simulink model "MVDR_example_hdl_4x4_systolic"  (R2020a)
settings: Solver=FixedStepDiscrete  StartTime=0.0  StopTime=stoptime  RelTol=1e-3
InitFcn:
  | model_init
values from neighbouring files (symbols this model uses):
  BackSubstitutePrototype = fi(0, matrixdivbacksub_dt)    [model_init.m]
  matrixDivDelay = NumberOfCORDICIterations*10 + 86    [model_init.m]
  movavg_bitshift = nextpow2(sqrt(windowSize))    [model_init.m]
  mvdrPipelineDelay = covMatDelay+movAvgDelay+matrixDivDelay+normResponseDelay    [model_init.m]
  numArrayElements = 4    [model_init.m]
  NumberOfCORDICIterations = matrixdivin_dt.WordLength - 1    [model_init.m]
  srcAngles = [20 60]    [model_init.m]
  sv = step(steeringVector,fc,[scanAngle; 0])    [model_init.m]
  Ts = 1/fs    (= 7.8125e-09)    [model_init.m]
  windowSize = 1024    [model_init.m]
libraries: hdlsllib x249, simulink x44, commfilt2 x4, commrfcorlib x3, commsync2 x3, commrflib2 x2, commrandsrc3 x2, phasedtxrxlib x2, commdigbbndcpm2 x1, dspsolvers x1, embreciprocals x1, commdigbbndpm3 x1
(part 6 of 11)

== system MVDR_example_hdl_4x4_systolic/MVDR HDL/Compute Weight Vector/Matrix Left Divide/CORDIC/4x4 Complex CORDIC Matrix Left Divide/Q'B, R 4x4 Complex CORDIC Systolic Array/Leading Complex Row Rotation - 4/Rotate first element to real - 1 ==
  x : Inport
  u : Inport  Port=2
  validIn : Inport  Port=3
  Complex to Real-Imag : ComplexToRealImag
  Complex to Real-Imag1 : ComplexToRealImag
  Delay{4..7,9..10,15} (7 alike) : Delay  DelayLength=1
  Force imaginary part to exactly zero : MATLAB Function  TreatAsAtomicUnit=on
  Inverse CORDIC Gain1 : Subsystem  TreatAsAtomicUnit=on  mask{NumberOfCORDICIterations=NumberOfCORDICIterations}
      mask prompts: NumberOfCORDICIterations "Number of CORDIC Iterations"
      mask Display: disp('1/An')
  Inverse CORDIC Gain2 : Subsystem  TreatAsAtomicUnit=on  mask{NumberOfCORDICIterations=NumberOfCORDICIterations}
      mask prompts: NumberOfCORDICIterations "Number of CORDIC Iterations"
      mask Display: disp('1/An')
  Inverse CORDIC Gain3 : Subsystem  TreatAsAtomicUnit=on  mask{NumberOfCORDICIterations=NumberOfCORDICIterations}
      mask prompts: NumberOfCORDICIterations "Number of CORDIC Iterations"
      mask Display: disp('1/An')
  Inverse CORDIC Gain4 : Subsystem  TreatAsAtomicUnit=on  mask{NumberOfCORDICIterations=NumberOfCORDICIterations}
      mask prompts: NumberOfCORDICIterations "Number of CORDIC Iterations"
      mask Display: disp('1/An')
  "Q'B, R Row Rotations - Real" : Subsystem  TreatAsAtomicUnit=on  mask{NumberOfCORDICIterations=NumberOfCORDICIterations}
      mask prompts: NumberOfCORDICIterations "Number of CORDIC Iterations"
  QR 3rd and 4th Quadrant Compensation : MATLAB Function  TreatAsAtomicUnit=on
  Real-Imag to Complex : RealImagToComplex
  Real-Imag to Complex1 : RealImagToComplex
  State Control : StateControl  StateControl=Synchronous
  Unit Delay Enabled Synchronous{,1..3} (4 alike) : hdlsllib/Discrete/Unit Delay Enabled Synchronous  InitialCondition=0.0  SampleTime=-1
      settings: SourceProductBaseCode=SL
  ValidIn to Ready Logic with Delay : Subsystem
  x' : Outport  VectorParamsAs1DForOutWhenUnconnected=off
  u' : Outport  Port=2  VectorParamsAs1DForOutWhenUnconnected=off
  validOut : Outport  Port=3  VectorParamsAs1DForOutWhenUnconnected=off
  ready : Outport  Port=4  VectorParamsAs1DForOutWhenUnconnected=off
  wires:
  Unit Delay Enabled Synchronous3/1 -> x'/1
  Real-Imag to Complex/1 -> Unit Delay Enabled Synchronous3/1
  Unit Delay Enabled Synchronous2/1 -> u'/1
  Real-Imag to Complex1/1 -> Unit Delay Enabled Synchronous2/1
  Unit Delay Enabled Synchronous1/1 -> Complex to Real-Imag/1
  Unit Delay Enabled Synchronous/1 -> Complex to Real-Imag1/1
  "Q'B, R Row Rotations - Real"/6(ready) -> ValidIn to Ready Logic with Delay/1(readyIn)
  ValidIn to Ready Logic with Delay/1(readyOut) -> ready/1
  Delay15/1 -> validOut/1
  "Q'B, R Row Rotations - Real"/5(validOut) -> Delay15/1, Unit Delay Enabled Synchronous3/2, Unit Delay Enabled Synchronous2/2
  Inverse CORDIC Gain3/1(Out1) -> Real-Imag to Complex1/2
  Inverse CORDIC Gain2/1(Out1) -> Real-Imag to Complex1/1
  Inverse CORDIC Gain1/1(Out1) -> Force imaginary part to exactly zero/1(u)
  Inverse CORDIC Gain4/1(Out1) -> Real-Imag to Complex/1
  Delay10/1 -> "Q'B, R Row Rotations - Real"/5(validIn), ValidIn to Ready Logic with Delay/2(validIn * z^-1)
  validIn/1 -> Delay9/1, Unit Delay Enabled Synchronous1/2, Unit Delay Enabled Synchronous/2
  Delay9/1 -> Delay10/1, ValidIn to Ready Logic with Delay/3(validIn)
  Force imaginary part to exactly zero/1(y) -> Real-Imag to Complex/2
  "Q'B, R Row Rotations - Real"/2(y_out) -> Inverse CORDIC Gain1/1(In1)
  u/1 -> Unit Delay Enabled Synchronous/1
  x/1 -> Unit Delay Enabled Synchronous1/1
  "Q'B, R Row Rotations - Real"/4(v_out) -> Inverse CORDIC Gain3/1(In1)
  "Q'B, R Row Rotations - Real"/3(u_out) -> Inverse CORDIC Gain2/1(In1)
  "Q'B, R Row Rotations - Real"/1(x_out) -> Inverse CORDIC Gain4/1(In1)
  Delay7/1 -> "Q'B, R Row Rotations - Real"/4(v)
  Delay6/1 -> "Q'B, R Row Rotations - Real"/3(u)
  Delay5/1 -> "Q'B, R Row Rotations - Real"/2(y)
  Delay4/1 -> "Q'B, R Row Rotations - Real"/1(x)
  Complex to Real-Imag1/2 -> QR 3rd and 4th Quadrant Compensation/4(v)
  Complex to Real-Imag1/1 -> QR 3rd and 4th Quadrant Compensation/3(u)
  Complex to Real-Imag/2 -> QR 3rd and 4th Quadrant Compensation/2(y)
  Complex to Real-Imag/1 -> QR 3rd and 4th Quadrant Compensation/1(x)
  QR 3rd and 4th Quadrant Compensation/4(v_out) -> Delay7/1
  QR 3rd and 4th Quadrant Compensation/2(y_out) -> Delay5/1
  QR 3rd and 4th Quadrant Compensation/3(u_out) -> Delay6/1
  QR 3rd and 4th Quadrant Compensation/1(x_out) -> Delay4/1

== system MVDR_example_hdl_4x4_systolic/MVDR HDL/Compute Weight Vector/Matrix Left Divide/CORDIC/4x4 Complex CORDIC Matrix Left Divide/Q'B, R 4x4 Complex CORDIC Systolic Array/Leading Complex Row Rotation - 4/ValidIn to Ready Logic ==
  readyIn : Inport
  validIn : Inport  Port=2
  AND : Logic  IconShape=distinctive  AllPortsSameDT=off  OutDataTypeStr=boolean
  NOT : Logic  Operator=NOT  IconShape=distinctive  AllPortsSameDT=off  OutDataTypeStr=boolean
  readyOut : Outport  VectorParamsAs1DForOutWhenUnconnected=off
  wires:
  validIn/1 -> NOT/1
  readyIn/1 -> AND/1
  AND/1 -> readyOut/1
  NOT/1 -> AND/2

== system MVDR_example_hdl_4x4_systolic/MVDR HDL/Compute Weight Vector/Matrix Left Divide/CORDIC/4x4 Complex CORDIC Matrix Left Divide/Q'B, R 4x4 Complex CORDIC Systolic Array/Leading Complex Row Rotation - 4/ValidIn to Ready Logic1 ==
  readyIn : Inport
  validIn : Inport  Port=2
  AND : Logic  IconShape=distinctive  AllPortsSameDT=off  OutDataTypeStr=boolean
  NOT : Logic  Operator=NOT  IconShape=distinctive  AllPortsSameDT=off  OutDataTypeStr=boolean
  readyOut : Outport  VectorParamsAs1DForOutWhenUnconnected=off
  wires:
  validIn/1 -> NOT/1
  readyIn/1 -> AND/1
  AND/1 -> readyOut/1
  NOT/1 -> AND/2

== system MVDR_example_hdl_4x4_systolic/MVDR HDL/Compute Weight Vector/Matrix Left Divide/CORDIC/4x4 Complex CORDIC Matrix Left Divide/Q'B, R 4x4 Complex CORDIC Systolic Array/Rotate first element to real/Inverse CORDIC Gain1 ==
  In1 : Inport
  Inverse CORDIC Gain : Gain  Gain=1/prod(sqrt(1+2.^(-2*(0:double(NumberOfCORDICIterations)-1))))  OutDataTypeStr=Inherit: Same as input
  Out1 : Outport  VectorParamsAs1DForOutWhenUnconnected=off
  wires:
  Inverse CORDIC Gain/1 -> Out1/1
  In1/1 -> Inverse CORDIC Gain/1

== system MVDR_example_hdl_4x4_systolic/MVDR HDL/Compute Weight Vector/Matrix Left Divide/CORDIC/4x4 Complex CORDIC Matrix Left Divide/Q'B, R 4x4 Complex CORDIC Systolic Array/Rotate first element to real/Inverse CORDIC Gain2 ==
  In1 : Inport
  Inverse CORDIC Gain : Gain  Gain=1/prod(sqrt(1+2.^(-2*(0:double(NumberOfCORDICIterations)-1))))  OutDataTypeStr=Inherit: Same as input
  Out1 : Outport  VectorParamsAs1DForOutWhenUnconnected=off
  wires:
  Inverse CORDIC Gain/1 -> Out1/1
  In1/1 -> Inverse CORDIC Gain/1

== system MVDR_example_hdl_4x4_systolic/MVDR HDL/Compute Weight Vector/Matrix Left Divide/CORDIC/4x4 Complex CORDIC Matrix Left Divide/Q'B, R 4x4 Complex CORDIC Systolic Array/Rotate first element to real/Inverse CORDIC Gain3 ==
  In1 : Inport
  Inverse CORDIC Gain : Gain  Gain=1/prod(sqrt(1+2.^(-2*(0:double(NumberOfCORDICIterations)-1))))  OutDataTypeStr=Inherit: Same as input
  Out1 : Outport  VectorParamsAs1DForOutWhenUnconnected=off
  wires:
  Inverse CORDIC Gain/1 -> Out1/1
  In1/1 -> Inverse CORDIC Gain/1

== system MVDR_example_hdl_4x4_systolic/MVDR HDL/Compute Weight Vector/Matrix Left Divide/CORDIC/4x4 Complex CORDIC Matrix Left Divide/Q'B, R 4x4 Complex CORDIC Systolic Array/Rotate first element to real/Inverse CORDIC Gain4 ==
  In1 : Inport
  Inverse CORDIC Gain : Gain  Gain=1/prod(sqrt(1+2.^(-2*(0:double(NumberOfCORDICIterations)-1))))  OutDataTypeStr=Inherit: Same as input
  Out1 : Outport  VectorParamsAs1DForOutWhenUnconnected=off
  wires:
  Inverse CORDIC Gain/1 -> Out1/1
  In1/1 -> Inverse CORDIC Gain/1

== system MVDR_example_hdl_4x4_systolic/MVDR HDL/Compute Weight Vector/Matrix Left Divide/CORDIC/4x4 Complex CORDIC Matrix Left Divide/Q'B, R 4x4 Complex CORDIC Systolic Array/Rotate first element to real/Q'B, R Row Rotations - Real ==
  x : Inport
  y : Inport  Port=2
  u : Inport  Port=3
  v : Inport  Port=4
  validIn : Inport  Port=5
  CORDIC Counter : Subsystem  mask{NumberOfCORDICIterations=NumberOfCORDICIterations}
      mask prompts: NumberOfCORDICIterations "Number of CORDIC Iterations"
  Delay{1..12} (12 alike) : Delay  DelayLength=1
  Delay13 : Delay  DelayLength=1  InitialCondition=true
  MATLAB Function : MATLAB Function  TreatAsAtomicUnit=on
  Same Datatype : Subsystem  TreatAsAtomicUnit=on
  Same Datatype1 : Subsystem  TreatAsAtomicUnit=on
  Same Datatype2 : Subsystem  TreatAsAtomicUnit=on
  Same Datatype3 : Subsystem  TreatAsAtomicUnit=on
  State Control : StateControl  StateControl=Synchronous
  Switch{,1..3} (4 alike) : Switch  Criteria=u2 ~= 0
  x_out : Outport  VectorParamsAs1DForOutWhenUnconnected=off
  y_out : Outport  Port=2  VectorParamsAs1DForOutWhenUnconnected=off
  u_out : Outport  Port=3  VectorParamsAs1DForOutWhenUnconnected=off
  v_out : Outport  Port=4  VectorParamsAs1DForOutWhenUnconnected=off
  validOut : Outport  Port=5  VectorParamsAs1DForOutWhenUnconnected=off
  ready : Outport  Port=6  VectorParamsAs1DForOutWhenUnconnected=off
  wires:
  Delay13/1 -> ready/1
  Delay12/1 -> Delay3/1
  Delay10/1 -> MATLAB Function/5(iteration)
  Delay9/1 -> Switch/2, Switch1/2, Switch2/2, Switch3/2
  Delay8/1 -> Same Datatype2/2(Reference), Switch3/3
  Delay6/1 -> Same Datatype3/2(Reference), Switch2/3
  Delay5/1 -> Same Datatype1/2(Reference), Switch1/3
  Delay4/1 -> Same Datatype/2(Reference), Switch/3
  Delay1/1 -> Same Datatype/1(Data), x_out/1
  Delay2/1 -> Same Datatype1/1(Data), y_out/1
  Delay11/1 -> Same Datatype2/1(Data), v_out/1
  MATLAB Function/1(x_out) -> Delay1/1
  MATLAB Function/2(y_out) -> Delay2/1
  MATLAB Function/3(u_out) -> Delay7/1
  MATLAB Function/4(v_out) -> Delay11/1
  Delay7/1 -> Same Datatype3/1(Data), u_out/1
  Delay3/1 -> validOut/1
  validIn/1 -> CORDIC Counter/1(validIn)
  CORDIC Counter/2(count) -> Delay10/1
  CORDIC Counter/3(last) -> Delay12/1
  CORDIC Counter/4(ready) -> Delay13/1
  Switch/1 -> MATLAB Function/1(x)
  Switch1/1 -> MATLAB Function/2(y)
  Switch2/1 -> MATLAB Function/3(u)
  Switch3/1 -> MATLAB Function/4(v)
  CORDIC Counter/1(count_is_positive) -> Delay9/1
  x/1 -> Delay4/1
  y/1 -> Delay5/1
  u/1 -> Delay6/1
  v/1 -> Delay8/1
  Same Datatype/1(DataOut) -> Switch/1
  Same Datatype1/1(DataOut) -> Switch1/1
  Same Datatype3/1(DataOut) -> Switch2/1
  Same Datatype2/1(DataOut) -> Switch3/1

== system MVDR_example_hdl_4x4_systolic/MVDR HDL/Compute Weight Vector/Matrix Left Divide/CORDIC/4x4 Complex CORDIC Matrix Left Divide/Q'B, R 4x4 Complex CORDIC Systolic Array/Rotate first element to real/ValidIn to Ready Logic with Delay ==
  readyIn : Inport
  validIn * z^-1 : Inport  Port=2
  validIn : Inport  Port=3
  AND : Logic  IconShape=distinctive  AllPortsSameDT=off  OutDataTypeStr=boolean
  AND1 : Logic  IconShape=distinctive  AllPortsSameDT=off  OutDataTypeStr=boolean
  NOT : Logic  Operator=NOT  IconShape=distinctive  AllPortsSameDT=off  OutDataTypeStr=boolean
  NOT1 : Logic  Operator=NOT  IconShape=distinctive  AllPortsSameDT=off  OutDataTypeStr=boolean
  readyOut : Outport  VectorParamsAs1DForOutWhenUnconnected=off
  wires:
  validIn * z^-1/1 -> NOT/1
  validIn/1 -> NOT1/1
  readyIn/1 -> AND/1
  AND1/1 -> readyOut/1
  NOT1/1 -> AND1/2
  NOT/1 -> AND/2
  AND/1 -> AND1/1

== system MVDR_example_hdl_4x4_systolic/MVDR HDL/Compute Weight Vector/Matrix Left Divide/CORDIC/4x4 Complex CORDIC Matrix Left Divide/Back Substitute 4x4 Complex CORDIC/Invert first element - Folded/CORDIC Reciprocal Normalized, Folded/CORDIC Reciprocal Rotations- Folded ==
  x_in : Inport
  validIn : Inport  Port=2
  CORDIC Counter : Subsystem  mask{NumberOfCORDICIterations=NumberOfCORDICIterations}
      mask prompts: NumberOfCORDICIterations "Number of CORDIC Iterations"
  CORDIC Divide Kernel : MATLAB Function  TreatAsAtomicUnit=on
  Delay{1..8} (8 alike) : Delay  DelayLength=1
  Same Datatype1 : Subsystem  TreatAsAtomicUnit=on
  Same Datatype2 : Subsystem  TreatAsAtomicUnit=on
  Same Datatype3 : Subsystem  TreatAsAtomicUnit=on
  z_out : Outport  VectorParamsAs1DForOutWhenUnconnected=off
  validOut : Outport  Port=2  VectorParamsAs1DForOutWhenUnconnected=off
  ready : Outport  Port=3  VectorParamsAs1DForOutWhenUnconnected=off
  wires:
  Delay1/1 -> Same Datatype2/1(Data)
  Delay2/1 -> Same Datatype1/1(Data)
  Delay7/1 -> Same Datatype3/1(Data), z_out/1
  validIn/1 -> CORDIC Counter/1(validIn)
  CORDIC Counter/1(count_is_positive) -> Delay4/1
  CORDIC Counter/2(count) -> Delay5/1
  CORDIC Divide Kernel/1(x_out) -> Delay1/1
  CORDIC Divide Kernel/2(y_out) -> Delay2/1
  CORDIC Divide Kernel/3(z_out) -> Delay7/1
  x_in/1 -> Delay3/1
  Same Datatype1/1(DataOut) -> CORDIC Divide Kernel/2(y_reg)
  Same Datatype3/1(DataOut) -> CORDIC Divide Kernel/3(z_reg)
  CORDIC Counter/3(last) -> Delay6/1
  Same Datatype2/1(DataOut) -> CORDIC Divide Kernel/1(x_reg)
  CORDIC Counter/4(ready) -> Delay8/1
  Delay3/1 -> Same Datatype3/2(Reference), Same Datatype1/2(Reference), Same Datatype2/2(Reference), CORDIC Divide Kernel/4(x_in)
  Delay4/1 -> CORDIC Divide Kernel/5(count_is_positive)
  Delay5/1 -> CORDIC Divide Kernel/6(iteration)
  Delay6/1 -> validOut/1
  Delay8/1 -> ready/1

== system MVDR_example_hdl_4x4_systolic/MVDR HDL/Compute Weight Vector/Matrix Left Divide/CORDIC/4x4 Complex CORDIC Matrix Left Divide/Back Substitute 4x4 Complex CORDIC/Invert first element - Folded/CORDIC Reciprocal Normalized, Folded/Normalizer ==
  u : Inport
  validIn : Inport  Port=2
  Delay{,1..5} (6 alike) : Delay  DelayLength=1
  normalizer_block : MATLAB Function  TreatAsAtomicUnit=on
  u_normalized : Outport  VectorParamsAs1DForOutWhenUnconnected=off
  is_negative : Outport  Port=2  VectorParamsAs1DForOutWhenUnconnected=off
  shift_amount : Outport  Port=3  VectorParamsAs1DForOutWhenUnconnected=off
  validOut : Outport  Port=4  VectorParamsAs1DForOutWhenUnconnected=off
  wires:
  Delay5/1 -> is_negative/1
  normalizer_block/2(is_negative) -> Delay5/1
  Delay4/1 -> validOut/1
  Delay3/1 -> Delay4/1
  validIn/1 -> Delay3/1
  Delay/1 -> normalizer_block/1(u)
  Delay2/1 -> shift_amount/1
  normalizer_block/1(u_normalized) -> Delay1/1
  Delay1/1 -> u_normalized/1
  u/1 -> Delay/1
  normalizer_block/3(shift_amount) -> Delay2/1

== system MVDR_example_hdl_4x4_systolic/MVDR HDL/Compute Weight Vector/Matrix Left Divide/CORDIC/4x4 Complex CORDIC Matrix Left Divide/Back Substitute 4x4 Complex CORDIC/Invert first element - Folded/CORDIC Reciprocal Normalized, Folded/ValidIn to Ready Logic ==
  readyIn : Inport
  validIn : Inport  Port=2
  AND : Logic  IconShape=distinctive  AllPortsSameDT=off  OutDataTypeStr=boolean
  NOT : Logic  Operator=NOT  IconShape=distinctive  AllPortsSameDT=off  OutDataTypeStr=boolean
  readyOut : Outport  VectorParamsAs1DForOutWhenUnconnected=off
  wires:
  validIn/1 -> NOT/1
  readyIn/1 -> AND/1
  AND/1 -> readyOut/1
  NOT/1 -> AND/2

== system MVDR_example_hdl_4x4_systolic/MVDR HDL/Compute Weight Vector/Matrix Left Divide/CORDIC/4x4 Complex CORDIC Matrix Left Divide/Back Substitute 4x4 Complex CORDIC/Invert first element - Folded/CORDIC Reciprocal Normalized, Folded/ValidIn to Ready Logic1 ==
  readyIn : Inport
  validIn : Inport  Port=2
  AND : Logic  IconShape=distinctive  AllPortsSameDT=off  OutDataTypeStr=boolean
  NOT : Logic  Operator=NOT  IconShape=distinctive  AllPortsSameDT=off  OutDataTypeStr=boolean
  readyOut : Outport  VectorParamsAs1DForOutWhenUnconnected=off
  wires:
  validIn/1 -> NOT/1
  readyIn/1 -> AND/1
  AND/1 -> readyOut/1
  NOT/1 -> AND/2

== system MVDR_example_hdl_4x4_systolic/MVDR HDL/Compute Weight Vector/Matrix Left Divide/CORDIC/4x4 Complex CORDIC Matrix Left Divide/Back Substitute 4x4 Complex CORDIC/Invert first element - Folded/CORDIC Reciprocal Normalized, Folded/ValidIn to Ready Logic2 ==
  readyIn : Inport
  validIn : Inport  Port=2
  AND : Logic  IconShape=distinctive  AllPortsSameDT=off  OutDataTypeStr=boolean
  NOT : Logic  Operator=NOT  IconShape=distinctive  AllPortsSameDT=off  OutDataTypeStr=boolean
  readyOut : Outport  VectorParamsAs1DForOutWhenUnconnected=off
  wires:
  validIn/1 -> NOT/1
  readyIn/1 -> AND/1
  AND/1 -> readyOut/1
  NOT/1 -> AND/2

== system MVDR_example_hdl_4x4_systolic/MVDR HDL/Compute Weight Vector/Matrix Left Divide/CORDIC/4x4 Complex CORDIC Matrix Left Divide/Back Substitute 4x4 Complex CORDIC/Invert first element - Folded1/CORDIC Reciprocal Normalized, Folded/CORDIC Reciprocal Rotations- Folded ==
  x_in : Inport
  validIn : Inport  Port=2
  CORDIC Counter : Subsystem  mask{NumberOfCORDICIterations=NumberOfCORDICIterations}
      mask prompts: NumberOfCORDICIterations "Number of CORDIC Iterations"
  CORDIC Divide Kernel : MATLAB Function  TreatAsAtomicUnit=on
  Delay{1..8} (8 alike) : Delay  DelayLength=1
  Same Datatype1 : Subsystem  TreatAsAtomicUnit=on
  Same Datatype2 : Subsystem  TreatAsAtomicUnit=on
  Same Datatype3 : Subsystem  TreatAsAtomicUnit=on
  z_out : Outport  VectorParamsAs1DForOutWhenUnconnected=off
  validOut : Outport  Port=2  VectorParamsAs1DForOutWhenUnconnected=off
  ready : Outport  Port=3  VectorParamsAs1DForOutWhenUnconnected=off
  wires:
  Delay8/1 -> ready/1
  Delay6/1 -> validOut/1
  Delay5/1 -> CORDIC Divide Kernel/6(iteration)
  Delay4/1 -> CORDIC Divide Kernel/5(count_is_positive)
  Delay3/1 -> CORDIC Divide Kernel/4(x_in), Same Datatype2/2(Reference), Same Datatype1/2(Reference), Same Datatype3/2(Reference)
  CORDIC Counter/4(ready) -> Delay8/1
  Same Datatype2/1(DataOut) -> CORDIC Divide Kernel/1(x_reg)
  CORDIC Counter/3(last) -> Delay6/1
  Same Datatype3/1(DataOut) -> CORDIC Divide Kernel/3(z_reg)
  Same Datatype1/1(DataOut) -> CORDIC Divide Kernel/2(y_reg)
  x_in/1 -> Delay3/1
  CORDIC Divide Kernel/3(z_out) -> Delay7/1
  CORDIC Divide Kernel/2(y_out) -> Delay2/1
  CORDIC Divide Kernel/1(x_out) -> Delay1/1
  CORDIC Counter/2(count) -> Delay5/1
  CORDIC Counter/1(count_is_positive) -> Delay4/1
  validIn/1 -> CORDIC Counter/1(validIn)
  Delay7/1 -> z_out/1, Same Datatype3/1(Data)
  Delay2/1 -> Same Datatype1/1(Data)
  Delay1/1 -> Same Datatype2/1(Data)

== system MVDR_example_hdl_4x4_systolic/MVDR HDL/Compute Weight Vector/Matrix Left Divide/CORDIC/4x4 Complex CORDIC Matrix Left Divide/Back Substitute 4x4 Complex CORDIC/Invert first element - Folded1/CORDIC Reciprocal Normalized, Folded/Normalizer ==
  u : Inport
  validIn : Inport  Port=2
  Delay{,1..5} (6 alike) : Delay  DelayLength=1
  normalizer_block : MATLAB Function  TreatAsAtomicUnit=on
  u_normalized : Outport  VectorParamsAs1DForOutWhenUnconnected=off
  is_negative : Outport  Port=2  VectorParamsAs1DForOutWhenUnconnected=off
  shift_amount : Outport  Port=3  VectorParamsAs1DForOutWhenUnconnected=off
  validOut : Outport  Port=4  VectorParamsAs1DForOutWhenUnconnected=off
  wires:
  Delay5/1 -> is_negative/1
  normalizer_block/2(is_negative) -> Delay5/1
  Delay4/1 -> validOut/1
  Delay3/1 -> Delay4/1
  validIn/1 -> Delay3/1
  Delay/1 -> normalizer_block/1(u)
  Delay2/1 -> shift_amount/1
  normalizer_block/1(u_normalized) -> Delay1/1
  Delay1/1 -> u_normalized/1
  u/1 -> Delay/1
  normalizer_block/3(shift_amount) -> Delay2/1

== system MVDR_example_hdl_4x4_systolic/MVDR HDL/Compute Weight Vector/Matrix Left Divide/CORDIC/4x4 Complex CORDIC Matrix Left Divide/Back Substitute 4x4 Complex CORDIC/Invert first element - Folded1/CORDIC Reciprocal Normalized, Folded/ValidIn to Ready Logic ==
  readyIn : Inport
  validIn : Inport  Port=2
  AND : Logic  IconShape=distinctive  AllPortsSameDT=off  OutDataTypeStr=boolean
  NOT : Logic  Operator=NOT  IconShape=distinctive  AllPortsSameDT=off  OutDataTypeStr=boolean
  readyOut : Outport  VectorParamsAs1DForOutWhenUnconnected=off
  wires:
  validIn/1 -> NOT/1
  readyIn/1 -> AND/1
  AND/1 -> readyOut/1
  NOT/1 -> AND/2

== system MVDR_example_hdl_4x4_systolic/MVDR HDL/Compute Weight Vector/Matrix Left Divide/CORDIC/4x4 Complex CORDIC Matrix Left Divide/Back Substitute 4x4 Complex CORDIC/Invert first element - Folded1/CORDIC Reciprocal Normalized, Folded/ValidIn to Ready Logic1 ==
  readyIn : Inport
  validIn : Inport  Port=2
  AND : Logic  IconShape=distinctive  AllPortsSameDT=off  OutDataTypeStr=boolean
  NOT : Logic  Operator=NOT  IconShape=distinctive  AllPortsSameDT=off  OutDataTypeStr=boolean
  readyOut : Outport  VectorParamsAs1DForOutWhenUnconnected=off
  wires:
  validIn/1 -> NOT/1
  readyIn/1 -> AND/1
  AND/1 -> readyOut/1
  NOT/1 -> AND/2

== system MVDR_example_hdl_4x4_systolic/MVDR HDL/Compute Weight Vector/Matrix Left Divide/CORDIC/4x4 Complex CORDIC Matrix Left Divide/Back Substitute 4x4 Complex CORDIC/Invert first element - Folded1/CORDIC Reciprocal Normalized, Folded/ValidIn to Ready Logic2 ==
  readyIn : Inport
  validIn : Inport  Port=2
  AND : Logic  IconShape=distinctive  AllPortsSameDT=off  OutDataTypeStr=boolean
  NOT : Logic  Operator=NOT  IconShape=distinctive  AllPortsSameDT=off  OutDataTypeStr=boolean
  readyOut : Outport  VectorParamsAs1DForOutWhenUnconnected=off
  wires:
  validIn/1 -> NOT/1
  readyIn/1 -> AND/1
  AND/1 -> readyOut/1
  NOT/1 -> AND/2

== system MVDR_example_hdl_4x4_systolic/MVDR HDL/Compute Weight Vector/Matrix Left Divide/CORDIC/4x4 Complex CORDIC Matrix Left Divide/Back Substitute 4x4 Complex CORDIC/Invert first element - Folded2/CORDIC Reciprocal Normalized, Folded/CORDIC Reciprocal Rotations- Folded ==
  x_in : Inport
  validIn : Inport  Port=2
  CORDIC Counter : Subsystem  mask{NumberOfCORDICIterations=NumberOfCORDICIterations}
      mask prompts: NumberOfCORDICIterations "Number of CORDIC Iterations"
  CORDIC Divide Kernel : MATLAB Function  TreatAsAtomicUnit=on
  Delay{1..8} (8 alike) : Delay  DelayLength=1
  Same Datatype1 : Subsystem  TreatAsAtomicUnit=on
  Same Datatype2 : Subsystem  TreatAsAtomicUnit=on
  Same Datatype3 : Subsystem  TreatAsAtomicUnit=on
  z_out : Outport  VectorParamsAs1DForOutWhenUnconnected=off
  validOut : Outport  Port=2  VectorParamsAs1DForOutWhenUnconnected=off
  ready : Outport  Port=3  VectorParamsAs1DForOutWhenUnconnected=off
  wires:
  Delay8/1 -> ready/1
  Delay6/1 -> validOut/1
  Delay5/1 -> CORDIC Divide Kernel/6(iteration)
  Delay4/1 -> CORDIC Divide Kernel/5(count_is_positive)
  Delay3/1 -> CORDIC Divide Kernel/4(x_in), Same Datatype2/2(Reference), Same Datatype1/2(Reference), Same Datatype3/2(Reference)
  CORDIC Counter/4(ready) -> Delay8/1
  Same Datatype2/1(DataOut) -> CORDIC Divide Kernel/1(x_reg)
  CORDIC Counter/3(last) -> Delay6/1
  Same Datatype3/1(DataOut) -> CORDIC Divide Kernel/3(z_reg)
  Same Datatype1/1(DataOut) -> CORDIC Divide Kernel/2(y_reg)
  x_in/1 -> Delay3/1
  CORDIC Divide Kernel/3(z_out) -> Delay7/1
  CORDIC Divide Kernel/2(y_out) -> Delay2/1
  CORDIC Divide Kernel/1(x_out) -> Delay1/1
  CORDIC Counter/2(count) -> Delay5/1
  CORDIC Counter/1(count_is_positive) -> Delay4/1
  validIn/1 -> CORDIC Counter/1(validIn)
  Delay7/1 -> z_out/1, Same Datatype3/1(Data)
  Delay2/1 -> Same Datatype1/1(Data)
  Delay1/1 -> Same Datatype2/1(Data)

== system MVDR_example_hdl_4x4_systolic/MVDR HDL/Compute Weight Vector/Matrix Left Divide/CORDIC/4x4 Complex CORDIC Matrix Left Divide/Back Substitute 4x4 Complex CORDIC/Invert first element - Folded2/CORDIC Reciprocal Normalized, Folded/Normalizer ==
  u : Inport
  validIn : Inport  Port=2
  Delay{,1..5} (6 alike) : Delay  DelayLength=1
  normalizer_block : MATLAB Function  TreatAsAtomicUnit=on
  u_normalized : Outport  VectorParamsAs1DForOutWhenUnconnected=off
  is_negative : Outport  Port=2  VectorParamsAs1DForOutWhenUnconnected=off
  shift_amount : Outport  Port=3  VectorParamsAs1DForOutWhenUnconnected=off
  validOut : Outport  Port=4  VectorParamsAs1DForOutWhenUnconnected=off
  wires:
  Delay5/1 -> is_negative/1
  normalizer_block/2(is_negative) -> Delay5/1
  Delay4/1 -> validOut/1
  Delay3/1 -> Delay4/1
  validIn/1 -> Delay3/1
  Delay/1 -> normalizer_block/1(u)
  Delay2/1 -> shift_amount/1
  normalizer_block/1(u_normalized) -> Delay1/1
  Delay1/1 -> u_normalized/1
  u/1 -> Delay/1
  normalizer_block/3(shift_amount) -> Delay2/1

== system MVDR_example_hdl_4x4_systolic/MVDR HDL/Compute Weight Vector/Matrix Left Divide/CORDIC/4x4 Complex CORDIC Matrix Left Divide/Back Substitute 4x4 Complex CORDIC/Invert first element - Folded2/CORDIC Reciprocal Normalized, Folded/ValidIn to Ready Logic ==
  readyIn : Inport
  validIn : Inport  Port=2
  AND : Logic  IconShape=distinctive  AllPortsSameDT=off  OutDataTypeStr=boolean
  NOT : Logic  Operator=NOT  IconShape=distinctive  AllPortsSameDT=off  OutDataTypeStr=boolean
  readyOut : Outport  VectorParamsAs1DForOutWhenUnconnected=off
  wires:
  validIn/1 -> NOT/1
  readyIn/1 -> AND/1
  AND/1 -> readyOut/1
  NOT/1 -> AND/2

== system MVDR_example_hdl_4x4_systolic/MVDR HDL/Compute Weight Vector/Matrix Left Divide/CORDIC/4x4 Complex CORDIC Matrix Left Divide/Back Substitute 4x4 Complex CORDIC/Invert first element - Folded2/CORDIC Reciprocal Normalized, Folded/ValidIn to Ready Logic1 ==
  readyIn : Inport
  validIn : Inport  Port=2
  AND : Logic  IconShape=distinctive  AllPortsSameDT=off  OutDataTypeStr=boolean
  NOT : Logic  Operator=NOT  IconShape=distinctive  AllPortsSameDT=off  OutDataTypeStr=boolean
  readyOut : Outport  VectorParamsAs1DForOutWhenUnconnected=off
  wires:
  validIn/1 -> NOT/1
  readyIn/1 -> AND/1
  AND/1 -> readyOut/1
  NOT/1 -> AND/2

== system MVDR_example_hdl_4x4_systolic/MVDR HDL/Compute Weight Vector/Matrix Left Divide/CORDIC/4x4 Complex CORDIC Matrix Left Divide/Back Substitute 4x4 Complex CORDIC/Invert first element - Folded2/CORDIC Reciprocal Normalized, Folded/ValidIn to Ready Logic2 ==
  readyIn : Inport
  validIn : Inport  Port=2
  AND : Logic  IconShape=distinctive  AllPortsSameDT=off  OutDataTypeStr=boolean
  NOT : Logic  Operator=NOT  IconShape=distinctive  AllPortsSameDT=off  OutDataTypeStr=boolean
  readyOut : Outport  VectorParamsAs1DForOutWhenUnconnected=off
  wires:
  validIn/1 -> NOT/1
  readyIn/1 -> AND/1
  AND/1 -> readyOut/1
  NOT/1 -> AND/2

== system MVDR_example_hdl_4x4_systolic/MVDR HDL/Compute Weight Vector/Matrix Left Divide/CORDIC/4x4 Complex CORDIC Matrix Left Divide/Back Substitute 4x4 Complex CORDIC/Invert first element - Folded3/CORDIC Reciprocal Normalized, Folded/CORDIC Reciprocal Rotations- Folded ==
  x_in : Inport
  validIn : Inport  Port=2
  CORDIC Counter : Subsystem  mask{NumberOfCORDICIterations=NumberOfCORDICIterations}
      mask prompts: NumberOfCORDICIterations "Number of CORDIC Iterations"
  CORDIC Divide Kernel : MATLAB Function  TreatAsAtomicUnit=on
  Delay{1..8} (8 alike) : Delay  DelayLength=1
  Same Datatype1 : Subsystem  TreatAsAtomicUnit=on
  Same Datatype2 : Subsystem  TreatAsAtomicUnit=on
  Same Datatype3 : Subsystem  TreatAsAtomicUnit=on
  z_out : Outport  VectorParamsAs1DForOutWhenUnconnected=off
  validOut : Outport  Port=2  VectorParamsAs1DForOutWhenUnconnected=off
  ready : Outport  Port=3  VectorParamsAs1DForOutWhenUnconnected=off
  wires:
  Delay8/1 -> ready/1
  Delay6/1 -> validOut/1
  Delay5/1 -> CORDIC Divide Kernel/6(iteration)
  Delay4/1 -> CORDIC Divide Kernel/5(count_is_positive)
  Delay3/1 -> CORDIC Divide Kernel/4(x_in), Same Datatype2/2(Reference), Same Datatype1/2(Reference), Same Datatype3/2(Reference)
  CORDIC Counter/4(ready) -> Delay8/1
  Same Datatype2/1(DataOut) -> CORDIC Divide Kernel/1(x_reg)
  CORDIC Counter/3(last) -> Delay6/1
  Same Datatype3/1(DataOut) -> CORDIC Divide Kernel/3(z_reg)
  Same Datatype1/1(DataOut) -> CORDIC Divide Kernel/2(y_reg)
  x_in/1 -> Delay3/1
  CORDIC Divide Kernel/3(z_out) -> Delay7/1
  CORDIC Divide Kernel/2(y_out) -> Delay2/1
  CORDIC Divide Kernel/1(x_out) -> Delay1/1
  CORDIC Counter/2(count) -> Delay5/1
  CORDIC Counter/1(count_is_positive) -> Delay4/1
  validIn/1 -> CORDIC Counter/1(validIn)
  Delay7/1 -> z_out/1, Same Datatype3/1(Data)
  Delay2/1 -> Same Datatype1/1(Data)
  Delay1/1 -> Same Datatype2/1(Data)

== system MVDR_example_hdl_4x4_systolic/MVDR HDL/Compute Weight Vector/Matrix Left Divide/CORDIC/4x4 Complex CORDIC Matrix Left Divide/Back Substitute 4x4 Complex CORDIC/Invert first element - Folded3/CORDIC Reciprocal Normalized, Folded/Normalizer ==
  u : Inport
  validIn : Inport  Port=2
  Delay{,1..5} (6 alike) : Delay  DelayLength=1
  normalizer_block : MATLAB Function  TreatAsAtomicUnit=on
  u_normalized : Outport  VectorParamsAs1DForOutWhenUnconnected=off
  is_negative : Outport  Port=2  VectorParamsAs1DForOutWhenUnconnected=off
  shift_amount : Outport  Port=3  VectorParamsAs1DForOutWhenUnconnected=off
  validOut : Outport  Port=4  VectorParamsAs1DForOutWhenUnconnected=off
  wires:
  Delay5/1 -> is_negative/1
  normalizer_block/2(is_negative) -> Delay5/1
  Delay4/1 -> validOut/1
  Delay3/1 -> Delay4/1
  validIn/1 -> Delay3/1
  Delay/1 -> normalizer_block/1(u)
  Delay2/1 -> shift_amount/1
  normalizer_block/1(u_normalized) -> Delay1/1
  Delay1/1 -> u_normalized/1
  u/1 -> Delay/1
  normalizer_block/3(shift_amount) -> Delay2/1

== system MVDR_example_hdl_4x4_systolic/MVDR HDL/Compute Weight Vector/Matrix Left Divide/CORDIC/4x4 Complex CORDIC Matrix Left Divide/Back Substitute 4x4 Complex CORDIC/Invert first element - Folded3/CORDIC Reciprocal Normalized, Folded/ValidIn to Ready Logic ==
  readyIn : Inport
  validIn : Inport  Port=2
  AND : Logic  IconShape=distinctive  AllPortsSameDT=off  OutDataTypeStr=boolean
  NOT : Logic  Operator=NOT  IconShape=distinctive  AllPortsSameDT=off  OutDataTypeStr=boolean
  readyOut : Outport  VectorParamsAs1DForOutWhenUnconnected=off
  wires:
  validIn/1 -> NOT/1
  readyIn/1 -> AND/1
  AND/1 -> readyOut/1
  NOT/1 -> AND/2

== system MVDR_example_hdl_4x4_systolic/MVDR HDL/Compute Weight Vector/Matrix Left Divide/CORDIC/4x4 Complex CORDIC Matrix Left Divide/Back Substitute 4x4 Complex CORDIC/Invert first element - Folded3/CORDIC Reciprocal Normalized, Folded/ValidIn to Ready Logic1 ==
  readyIn : Inport
  validIn : Inport  Port=2
  AND : Logic  IconShape=distinctive  AllPortsSameDT=off  OutDataTypeStr=boolean
  NOT : Logic  Operator=NOT  IconShape=distinctive  AllPortsSameDT=off  OutDataTypeStr=boolean
  readyOut : Outport  VectorParamsAs1DForOutWhenUnconnected=off
  wires:
  validIn/1 -> NOT/1
  readyIn/1 -> AND/1
  AND/1 -> readyOut/1
  NOT/1 -> AND/2

== system MVDR_example_hdl_4x4_systolic/MVDR HDL/Compute Weight Vector/Matrix Left Divide/CORDIC/4x4 Complex CORDIC Matrix Left Divide/Back Substitute 4x4 Complex CORDIC/Invert first element - Folded3/CORDIC Reciprocal Normalized, Folded/ValidIn to Ready Logic2 ==
  readyIn : Inport
  validIn : Inport  Port=2
  AND : Logic  IconShape=distinctive  AllPortsSameDT=off  OutDataTypeStr=boolean
  NOT : Logic  Operator=NOT  IconShape=distinctive  AllPortsSameDT=off  OutDataTypeStr=boolean
  readyOut : Outport  VectorParamsAs1DForOutWhenUnconnected=off
  wires:
  validIn/1 -> NOT/1
  readyIn/1 -> AND/1
  AND/1 -> readyOut/1
  NOT/1 -> AND/2

== system MVDR_example_hdl_4x4_systolic/MVDR HDL/Compute Weight Vector/Matrix Left Divide/CORDIC/4x4 Complex CORDIC Matrix Left Divide/Q'B, R 4x4 Complex CORDIC Systolic Array/Complex Row Rotation with real pivots/Q'B, R Row Rotations - Complex/CORDIC Counter ==
  validIn : Inport
  Compare To Constant : simulink/Logic and Bit Operations/Compare To Constant  relop===  const=NumberOfCORDICIterations-1  OutDataTypeStr=boolean
  Compare To Zero : simulink/Logic and Bit Operations/Compare To Zero  relop=>  OutDataTypeStr=boolean
  HDL Counter1 : hdlsllib/Sources/HDL Counter  CountType=Count limited  CountInit=0  CountStep=1  CountMax=NumberOfCORDICIterations-1  CountFromType=Initial value  CountFrom=0  CountResetPort=off  CountLoadPort=off  CountEnbPort=on  CountDirPort=off  CountDataType=Unsigned  CountWordLen=nextpow2(NumberOfCORDICIterations)  CountFracLen=0  CountSampTime=1
  OR : Logic  Operator=OR  IconShape=distinctive  AllPortsSameDT=off  OutDataTypeStr=boolean
  SR_latch : Subsystem
  State Control : StateControl  StateControl=Synchronous
  ValidIn to Ready Logic : Subsystem
  count_is_positive : Outport  VectorParamsAs1DForOutWhenUnconnected=off
  count : Outport  Port=2  VectorParamsAs1DForOutWhenUnconnected=off
  last : Outport  Port=3  VectorParamsAs1DForOutWhenUnconnected=off
  ready : Outport  Port=4  VectorParamsAs1DForOutWhenUnconnected=off
  wires:
  ValidIn to Ready Logic/1(readyOut) -> ready/1
  SR_latch/1(Q) -> ValidIn to Ready Logic/1(readyIn)  "ready"
  validIn/1 -> OR/2, SR_latch/2(R), ValidIn to Ready Logic/2(validIn)
  Compare To Constant/1 -> last/1, SR_latch/1(S)
  Compare To Zero/1 -> OR/1, count_is_positive/1
  OR/1 -> HDL Counter1/1
  HDL Counter1/1 -> Compare To Constant/1, count/1, Compare To Zero/1  "count"

== system MVDR_example_hdl_4x4_systolic/MVDR HDL/Compute Weight Vector/Matrix Left Divide/CORDIC/4x4 Complex CORDIC Matrix Left Divide/Q'B, R 4x4 Complex CORDIC Systolic Array/Complex Row Rotation with real pivots/Q'B, R Row Rotations - Complex/Same Datatype ==
  Data : Inport
  Reference : Inport  Port=2
  Data Type Duplicate : DataTypeDuplicate
  DataOut : Outport  VectorParamsAs1DForOutWhenUnconnected=off
  wires:
  Data/1 -> Data Type Duplicate/1, DataOut/1
  Reference/1 -> Data Type Duplicate/2

== system MVDR_example_hdl_4x4_systolic/MVDR HDL/Compute Weight Vector/Matrix Left Divide/CORDIC/4x4 Complex CORDIC Matrix Left Divide/Q'B, R 4x4 Complex CORDIC Systolic Array/Complex Row Rotation with real pivots/Q'B, R Row Rotations - Complex/Same Datatype1 ==
  Data : Inport
  Reference : Inport  Port=2
  Data Type Duplicate : DataTypeDuplicate
  DataOut : Outport  VectorParamsAs1DForOutWhenUnconnected=off
  wires:
  Data/1 -> Data Type Duplicate/1, DataOut/1
  Reference/1 -> Data Type Duplicate/2

== system MVDR_example_hdl_4x4_systolic/MVDR HDL/Compute Weight Vector/Matrix Left Divide/CORDIC/4x4 Complex CORDIC Matrix Left Divide/Q'B, R 4x4 Complex CORDIC Systolic Array/Complex Row Rotation with real pivots/Q'B, R Row Rotations - Complex/Same Datatype2 ==
  Data : Inport
  Reference : Inport  Port=2
  Data Type Duplicate : DataTypeDuplicate
  DataOut : Outport  VectorParamsAs1DForOutWhenUnconnected=off
  wires:
  Data/1 -> Data Type Duplicate/1, DataOut/1
  Reference/1 -> Data Type Duplicate/2

== system MVDR_example_hdl_4x4_systolic/MVDR HDL/Compute Weight Vector/Matrix Left Divide/CORDIC/4x4 Complex CORDIC Matrix Left Divide/Q'B, R 4x4 Complex CORDIC Systolic Array/Complex Row Rotation with real pivots/Q'B, R Row Rotations - Complex/Same Datatype3 ==
  Data : Inport
  Reference : Inport  Port=2
  Data Type Duplicate : DataTypeDuplicate
  DataOut : Outport  VectorParamsAs1DForOutWhenUnconnected=off
  wires:
  Data/1 -> Data Type Duplicate/1, DataOut/1
  Reference/1 -> Data Type Duplicate/2

== system MVDR_example_hdl_4x4_systolic/MVDR HDL/Compute Weight Vector/Matrix Left Divide/CORDIC/4x4 Complex CORDIC Matrix Left Divide/Q'B, R 4x4 Complex CORDIC Systolic Array/Complex Row Rotation 1/Q'B, R Row Rotations - Complex - Folded/CORDIC Counter ==
  validIn : Inport
  Compare To Constant : simulink/Logic and Bit Operations/Compare To Constant  relop===  const=NumberOfCORDICIterations-1  OutDataTypeStr=boolean
  Compare To Zero : simulink/Logic and Bit Operations/Compare To Zero  relop=>  OutDataTypeStr=boolean
  HDL Counter1 : hdlsllib/Sources/HDL Counter  CountType=Count limited  CountInit=0  CountStep=1  CountMax=NumberOfCORDICIterations-1  CountFromType=Initial value  CountFrom=0  CountResetPort=off  CountLoadPort=off  CountEnbPort=on  CountDirPort=off  CountDataType=Unsigned  CountWordLen=nextpow2(NumberOfCORDICIterations)  CountFracLen=0  CountSampTime=1
  OR : Logic  Operator=OR  IconShape=distinctive  AllPortsSameDT=off  OutDataTypeStr=boolean
  SR_latch : Subsystem
  State Control : StateControl  StateControl=Synchronous
  ValidIn to Ready Logic : Subsystem
  count_is_positive : Outport  VectorParamsAs1DForOutWhenUnconnected=off
  count : Outport  Port=2  VectorParamsAs1DForOutWhenUnconnected=off
  last : Outport  Port=3  VectorParamsAs1DForOutWhenUnconnected=off
  ready : Outport  Port=4  VectorParamsAs1DForOutWhenUnconnected=off
  wires:
  ValidIn to Ready Logic/1(readyOut) -> ready/1
  SR_latch/1(Q) -> ValidIn to Ready Logic/1(readyIn)  "ready"
  validIn/1 -> OR/2, SR_latch/2(R), ValidIn to Ready Logic/2(validIn)
  Compare To Constant/1 -> last/1, SR_latch/1(S)
  Compare To Zero/1 -> OR/1, count_is_positive/1
  OR/1 -> HDL Counter1/1
  HDL Counter1/1 -> Compare To Constant/1, count/1, Compare To Zero/1  "count"

== system MVDR_example_hdl_4x4_systolic/MVDR HDL/Compute Weight Vector/Matrix Left Divide/CORDIC/4x4 Complex CORDIC Matrix Left Divide/Q'B, R 4x4 Complex CORDIC Systolic Array/Complex Row Rotation 1/Q'B, R Row Rotations - Complex - Folded/Same Datatype ==
  Data : Inport
  Reference : Inport  Port=2
  Data Type Duplicate : DataTypeDuplicate
  DataOut : Outport  VectorParamsAs1DForOutWhenUnconnected=off
  wires:
  Data/1 -> Data Type Duplicate/1, DataOut/1
  Reference/1 -> Data Type Duplicate/2

== system MVDR_example_hdl_4x4_systolic/MVDR HDL/Compute Weight Vector/Matrix Left Divide/CORDIC/4x4 Complex CORDIC Matrix Left Divide/Q'B, R 4x4 Complex CORDIC Systolic Array/Complex Row Rotation 1/Q'B, R Row Rotations - Complex - Folded/Same Datatype1 ==
  Data : Inport
  Reference : Inport  Port=2
  Data Type Duplicate : DataTypeDuplicate
  DataOut : Outport  VectorParamsAs1DForOutWhenUnconnected=off
  wires:
  Data/1 -> Data Type Duplicate/1, DataOut/1
  Reference/1 -> Data Type Duplicate/2

== system MVDR_example_hdl_4x4_systolic/MVDR HDL/Compute Weight Vector/Matrix Left Divide/CORDIC/4x4 Complex CORDIC Matrix Left Divide/Q'B, R 4x4 Complex CORDIC Systolic Array/Complex Row Rotation 1/Q'B, R Row Rotations - Complex - Folded/Same Datatype2 ==
  Data : Inport
  Reference : Inport  Port=2
  Data Type Duplicate : DataTypeDuplicate
  DataOut : Outport  VectorParamsAs1DForOutWhenUnconnected=off
  wires:
  Data/1 -> Data Type Duplicate/1, DataOut/1
  Reference/1 -> Data Type Duplicate/2

== system MVDR_example_hdl_4x4_systolic/MVDR HDL/Compute Weight Vector/Matrix Left Divide/CORDIC/4x4 Complex CORDIC Matrix Left Divide/Q'B, R 4x4 Complex CORDIC Systolic Array/Complex Row Rotation 1/Q'B, R Row Rotations - Complex - Folded/Same Datatype3 ==
  Data : Inport
  Reference : Inport  Port=2
  Data Type Duplicate : DataTypeDuplicate
  DataOut : Outport  VectorParamsAs1DForOutWhenUnconnected=off
  wires:
  Data/1 -> Data Type Duplicate/1, DataOut/1
  Reference/1 -> Data Type Duplicate/2

== system MVDR_example_hdl_4x4_systolic/MVDR HDL/Compute Weight Vector/Matrix Left Divide/CORDIC/4x4 Complex CORDIC Matrix Left Divide/Q'B, R 4x4 Complex CORDIC Systolic Array/Complex Row Rotation 1/Rotate first element to real - Folded/Inverse CORDIC Gain1 ==
  In1 : Inport
  Inverse CORDIC Gain : Gain  Gain=1/prod(sqrt(1+2.^(-2*(0:double(NumberOfCORDICIterations)-1))))  OutDataTypeStr=Inherit: Same as input
  Out1 : Outport  VectorParamsAs1DForOutWhenUnconnected=off
  wires:
  Inverse CORDIC Gain/1 -> Out1/1
  In1/1 -> Inverse CORDIC Gain/1

== system MVDR_example_hdl_4x4_systolic/MVDR HDL/Compute Weight Vector/Matrix Left Divide/CORDIC/4x4 Complex CORDIC Matrix Left Divide/Q'B, R 4x4 Complex CORDIC Systolic Array/Complex Row Rotation 1/Rotate first element to real - Folded/Inverse CORDIC Gain2 ==
  In1 : Inport
  Inverse CORDIC Gain : Gain  Gain=1/prod(sqrt(1+2.^(-2*(0:double(NumberOfCORDICIterations)-1))))  OutDataTypeStr=Inherit: Same as input
  Out1 : Outport  VectorParamsAs1DForOutWhenUnconnected=off
  wires:
  Inverse CORDIC Gain/1 -> Out1/1
  In1/1 -> Inverse CORDIC Gain/1

== system MVDR_example_hdl_4x4_systolic/MVDR HDL/Compute Weight Vector/Matrix Left Divide/CORDIC/4x4 Complex CORDIC Matrix Left Divide/Q'B, R 4x4 Complex CORDIC Systolic Array/Complex Row Rotation 1/Rotate first element to real - Folded/Inverse CORDIC Gain3 ==
  In1 : Inport
  Inverse CORDIC Gain : Gain  Gain=1/prod(sqrt(1+2.^(-2*(0:double(NumberOfCORDICIterations)-1))))  OutDataTypeStr=Inherit: Same as input
  Out1 : Outport  VectorParamsAs1DForOutWhenUnconnected=off
  wires:
  Inverse CORDIC Gain/1 -> Out1/1
  In1/1 -> Inverse CORDIC Gain/1

== system MVDR_example_hdl_4x4_systolic/MVDR HDL/Compute Weight Vector/Matrix Left Divide/CORDIC/4x4 Complex CORDIC Matrix Left Divide/Q'B, R 4x4 Complex CORDIC Systolic Array/Complex Row Rotation 1/Rotate first element to real - Folded/Inverse CORDIC Gain4 ==
  In1 : Inport
  Inverse CORDIC Gain : Gain  Gain=1/prod(sqrt(1+2.^(-2*(0:double(NumberOfCORDICIterations)-1))))  OutDataTypeStr=Inherit: Same as input
  Out1 : Outport  VectorParamsAs1DForOutWhenUnconnected=off
  wires:
  Inverse CORDIC Gain/1 -> Out1/1
  In1/1 -> Inverse CORDIC Gain/1

== system MVDR_example_hdl_4x4_systolic/MVDR HDL/Compute Weight Vector/Matrix Left Divide/CORDIC/4x4 Complex CORDIC Matrix Left Divide/Q'B, R 4x4 Complex CORDIC Systolic Array/Complex Row Rotation 1/Rotate first element to real - Folded/Q'B, R Row Rotations - Real ==
  x : Inport
  y : Inport  Port=2
  u : Inport  Port=3
  v : Inport  Port=4
  validIn : Inport  Port=5
  CORDIC Counter : Subsystem  mask{NumberOfCORDICIterations=NumberOfCORDICIterations}
      mask prompts: NumberOfCORDICIterations "Number of CORDIC Iterations"
  Delay{1..12} (12 alike) : Delay  DelayLength=1
  Delay13 : Delay  DelayLength=1  InitialCondition=true
  MATLAB Function : MATLAB Function  TreatAsAtomicUnit=on
  Same Datatype : Subsystem  TreatAsAtomicUnit=on
  Same Datatype1 : Subsystem  TreatAsAtomicUnit=on
  Same Datatype2 : Subsystem  TreatAsAtomicUnit=on
  Same Datatype3 : Subsystem  TreatAsAtomicUnit=on
  State Control : StateControl  StateControl=Synchronous
  Switch{,1..3} (4 alike) : Switch  Criteria=u2 ~= 0
  x_out : Outport  VectorParamsAs1DForOutWhenUnconnected=off
  y_out : Outport  Port=2  VectorParamsAs1DForOutWhenUnconnected=off
  u_out : Outport  Port=3  VectorParamsAs1DForOutWhenUnconnected=off
  v_out : Outport  Port=4  VectorParamsAs1DForOutWhenUnconnected=off
  validOut : Outport  Port=5  VectorParamsAs1DForOutWhenUnconnected=off
  ready : Outport  Port=6  VectorParamsAs1DForOutWhenUnconnected=off
  wires:
  Same Datatype2/1(DataOut) -> Switch3/1
  Same Datatype3/1(DataOut) -> Switch2/1
  Same Datatype1/1(DataOut) -> Switch1/1
  Same Datatype/1(DataOut) -> Switch/1
  v/1 -> Delay8/1
  u/1 -> Delay6/1
  y/1 -> Delay5/1
  x/1 -> Delay4/1
  CORDIC Counter/1(count_is_positive) -> Delay9/1
  Switch3/1 -> MATLAB Function/4(v)
  Switch2/1 -> MATLAB Function/3(u)
  Switch1/1 -> MATLAB Function/2(y)
  Switch/1 -> MATLAB Function/1(x)
  CORDIC Counter/4(ready) -> Delay13/1
  CORDIC Counter/3(last) -> Delay12/1
  CORDIC Counter/2(count) -> Delay10/1
  validIn/1 -> CORDIC Counter/1(validIn)
  Delay3/1 -> validOut/1
  Delay7/1 -> u_out/1, Same Datatype3/1(Data)
  MATLAB Function/4(v_out) -> Delay11/1
  MATLAB Function/3(u_out) -> Delay7/1
  MATLAB Function/2(y_out) -> Delay2/1
  MATLAB Function/1(x_out) -> Delay1/1
  Delay11/1 -> v_out/1, Same Datatype2/1(Data)
  Delay2/1 -> y_out/1, Same Datatype1/1(Data)
  Delay1/1 -> x_out/1, Same Datatype/1(Data)
  Delay4/1 -> Switch/3, Same Datatype/2(Reference)
  Delay5/1 -> Switch1/3, Same Datatype1/2(Reference)
  Delay6/1 -> Switch2/3, Same Datatype3/2(Reference)
  Delay8/1 -> Switch3/3, Same Datatype2/2(Reference)
  Delay9/1 -> Switch3/2, Switch2/2, Switch1/2, Switch/2
  Delay10/1 -> MATLAB Function/5(iteration)
  Delay12/1 -> Delay3/1
  Delay13/1 -> ready/1

== system MVDR_example_hdl_4x4_systolic/MVDR HDL/Compute Weight Vector/Matrix Left Divide/CORDIC/4x4 Complex CORDIC Matrix Left Divide/Q'B, R 4x4 Complex CORDIC Systolic Array/Complex Row Rotation 1/Rotate first element to real - Folded/ValidIn to Ready Logic with Delay ==
  readyIn : Inport
  validIn * z^-1 : Inport  Port=2
  validIn : Inport  Port=3
  AND : Logic  IconShape=distinctive  AllPortsSameDT=off  OutDataTypeStr=boolean
  AND1 : Logic  IconShape=distinctive  AllPortsSameDT=off  OutDataTypeStr=boolean
  NOT : Logic  Operator=NOT  IconShape=distinctive  AllPortsSameDT=off  OutDataTypeStr=boolean
  NOT1 : Logic  Operator=NOT  IconShape=distinctive  AllPortsSameDT=off  OutDataTypeStr=boolean
  readyOut : Outport  VectorParamsAs1DForOutWhenUnconnected=off
  wires:
  validIn * z^-1/1 -> NOT/1
  validIn/1 -> NOT1/1
  readyIn/1 -> AND/1
  AND1/1 -> readyOut/1
  NOT1/1 -> AND1/2
  NOT/1 -> AND/2
  AND/1 -> AND1/1

== system MVDR_example_hdl_4x4_systolic/MVDR HDL/Compute Weight Vector/Matrix Left Divide/CORDIC/4x4 Complex CORDIC Matrix Left Divide/Q'B, R 4x4 Complex CORDIC Systolic Array/Leading Complex Row Rotation/Q'B, R Row Rotations - Complex/CORDIC Counter ==
  validIn : Inport
  Compare To Constant : simulink/Logic and Bit Operations/Compare To Constant  relop===  const=NumberOfCORDICIterations-1  OutDataTypeStr=boolean
  Compare To Zero : simulink/Logic and Bit Operations/Compare To Zero  relop=>  OutDataTypeStr=boolean
  HDL Counter1 : hdlsllib/Sources/HDL Counter  CountType=Count limited  CountInit=0  CountStep=1  CountMax=NumberOfCORDICIterations-1  CountFromType=Initial value  CountFrom=0  CountResetPort=off  CountLoadPort=off  CountEnbPort=on  CountDirPort=off  CountDataType=Unsigned  CountWordLen=nextpow2(NumberOfCORDICIterations)  CountFracLen=0  CountSampTime=1
  OR : Logic  Operator=OR  IconShape=distinctive  AllPortsSameDT=off  OutDataTypeStr=boolean
  SR_latch : Subsystem
  State Control : StateControl  StateControl=Synchronous
  ValidIn to Ready Logic : Subsystem
  count_is_positive : Outport  VectorParamsAs1DForOutWhenUnconnected=off
  count : Outport  Port=2  VectorParamsAs1DForOutWhenUnconnected=off
  last : Outport  Port=3  VectorParamsAs1DForOutWhenUnconnected=off
  ready : Outport  Port=4  VectorParamsAs1DForOutWhenUnconnected=off
  wires:
  ValidIn to Ready Logic/1(readyOut) -> ready/1
  SR_latch/1(Q) -> ValidIn to Ready Logic/1(readyIn)  "ready"
  validIn/1 -> OR/2, SR_latch/2(R), ValidIn to Ready Logic/2(validIn)
  Compare To Constant/1 -> last/1, SR_latch/1(S)
  Compare To Zero/1 -> OR/1, count_is_positive/1
  OR/1 -> HDL Counter1/1
  HDL Counter1/1 -> Compare To Constant/1, count/1, Compare To Zero/1  "count"

== system MVDR_example_hdl_4x4_systolic/MVDR HDL/Compute Weight Vector/Matrix Left Divide/CORDIC/4x4 Complex CORDIC Matrix Left Divide/Q'B, R 4x4 Complex CORDIC Systolic Array/Leading Complex Row Rotation/Q'B, R Row Rotations - Complex/Same Datatype ==
  Data : Inport
  Reference : Inport  Port=2
  Data Type Duplicate : DataTypeDuplicate
  DataOut : Outport  VectorParamsAs1DForOutWhenUnconnected=off
  wires:
  Data/1 -> Data Type Duplicate/1, DataOut/1
  Reference/1 -> Data Type Duplicate/2

== system MVDR_example_hdl_4x4_systolic/MVDR HDL/Compute Weight Vector/Matrix Left Divide/CORDIC/4x4 Complex CORDIC Matrix Left Divide/Q'B, R 4x4 Complex CORDIC Systolic Array/Leading Complex Row Rotation/Q'B, R Row Rotations - Complex/Same Datatype1 ==
  Data : Inport
  Reference : Inport  Port=2
  Data Type Duplicate : DataTypeDuplicate
  DataOut : Outport  VectorParamsAs1DForOutWhenUnconnected=off
  wires:
  Data/1 -> Data Type Duplicate/1, DataOut/1
  Reference/1 -> Data Type Duplicate/2

== system MVDR_example_hdl_4x4_systolic/MVDR HDL/Compute Weight Vector/Matrix Left Divide/CORDIC/4x4 Complex CORDIC Matrix Left Divide/Q'B, R 4x4 Complex CORDIC Systolic Array/Leading Complex Row Rotation/Q'B, R Row Rotations - Complex/Same Datatype2 ==
  Data : Inport
  Reference : Inport  Port=2
  Data Type Duplicate : DataTypeDuplicate
  DataOut : Outport  VectorParamsAs1DForOutWhenUnconnected=off
  wires:
  Data/1 -> Data Type Duplicate/1, DataOut/1
  Reference/1 -> Data Type Duplicate/2

== system MVDR_example_hdl_4x4_systolic/MVDR HDL/Compute Weight Vector/Matrix Left Divide/CORDIC/4x4 Complex CORDIC Matrix Left Divide/Q'B, R 4x4 Complex CORDIC Systolic Array/Leading Complex Row Rotation/Q'B, R Row Rotations - Complex/Same Datatype3 ==
  Data : Inport
  Reference : Inport  Port=2
  Data Type Duplicate : DataTypeDuplicate
  DataOut : Outport  VectorParamsAs1DForOutWhenUnconnected=off
  wires:
  Data/1 -> Data Type Duplicate/1, DataOut/1
  Reference/1 -> Data Type Duplicate/2

== system MVDR_example_hdl_4x4_systolic/MVDR HDL/Compute Weight Vector/Matrix Left Divide/CORDIC/4x4 Complex CORDIC Matrix Left Divide/Q'B, R 4x4 Complex CORDIC Systolic Array/Leading Complex Row Rotation/Rotate first element to real/Inverse CORDIC Gain1 ==
  In1 : Inport
  Inverse CORDIC Gain : Gain  Gain=1/prod(sqrt(1+2.^(-2*(0:double(NumberOfCORDICIterations)-1))))  OutDataTypeStr=Inherit: Same as input
  Out1 : Outport  VectorParamsAs1DForOutWhenUnconnected=off
  wires:
  Inverse CORDIC Gain/1 -> Out1/1
  In1/1 -> Inverse CORDIC Gain/1
